simulink model "dSPACE_discrete"  (Simulink 7.1)
settings: Solver=ode3  StartTime=0.0  StopTime=inf  FixedStep=0.0005  RelTol=1e-3
undefined symbols (not defined in the file): DiscIntNeverNeededParam
libraries: simulink x2
settings Model: Creator=Administrator  LastModifiedBy=Administrator

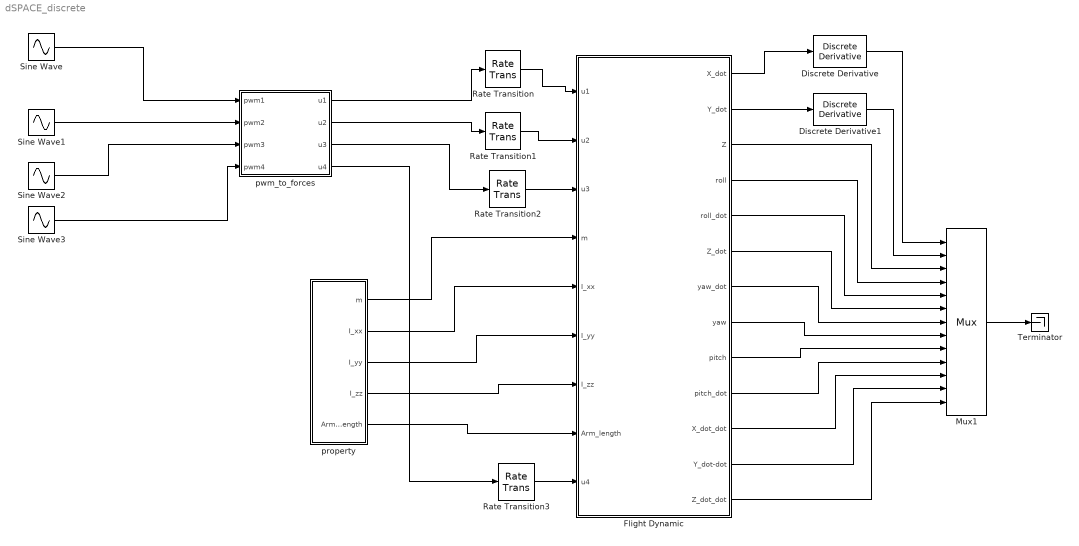
== system dSPACE_discrete ==
  Discrete Derivative : simulink/Discrete/Discrete Derivative  SystemSampleTime=-1  gainval=1.0  ICPrevScaledInput=0.0  OutMin=[]  OutMax=[]  OutDataType=sfix(16)  OutScaling=2^-10  DoSatur=off
  Discrete Derivative1 : simulink/Discrete/Discrete Derivative  SystemSampleTime=-1  gainval=1.0  ICPrevScaledInput=0.0  OutMin=[]  OutMax=[]  OutDataType=sfix(16)  OutScaling=2^-10  DoSatur=off
  Flight Dynamic : Subsystem
  Mux1 : Mux  Inputs=13
  Rate Transition{,1..3} (4 alike) : RateTransition
  Sine Wave{,1..3} (4 alike) : Sin  Amplitude=500  Bias=1500  SampleTime=0
  Terminator : Terminator
  "property " : Subsystem
  pwm_to_forces : Subsystem
  wires:
  Sine Wave1/1 -> pwm_to_forces/2(pwm2)
  Sine Wave2/1 -> pwm_to_forces/3(pwm3)
  Sine Wave3/1 -> pwm_to_forces/4(pwm4)
  Sine Wave/1 -> pwm_to_forces/1(pwm1)
  pwm_to_forces/1(u1) -> Rate Transition/1
  pwm_to_forces/2(u2) -> Rate Transition1/1
  pwm_to_forces/3(u3) -> Rate Transition2/1
  pwm_to_forces/4(u4) -> Rate Transition3/1
  "property "/1(m) -> Flight Dynamic/4(m)
  "property "/2(I_xx) -> Flight Dynamic/5(I_xx)
  "property "/3(I_yy) -> Flight Dynamic/6(I_yy)
  "property "/4(I_zz) -> Flight Dynamic/7(I_zz)
  "property "/5("Arm_length ") -> Flight Dynamic/8(Arm_length)
  Rate Transition/1 -> Flight Dynamic/1(u1)
  Rate Transition2/1 -> Flight Dynamic/3(u3)
  Rate Transition3/1 -> Flight Dynamic/9(u4)
  Rate Transition1/1 -> Flight Dynamic/2(u2)
  Flight Dynamic/1("X_dot ") -> Discrete Derivative/1
  Flight Dynamic/2(Y_dot) -> Discrete Derivative1/1
  Discrete Derivative/1 -> Mux1/1
  Discrete Derivative1/1 -> Mux1/2
  Flight Dynamic/3(Z) -> Mux1/3
  Flight Dynamic/4(roll) -> Mux1/4
  Flight Dynamic/5(roll_dot) -> Mux1/5
  Flight Dynamic/6(Z_dot) -> Mux1/6
  Flight Dynamic/7(yaw_dot) -> Mux1/7
  Flight Dynamic/8(yaw) -> Mux1/8
  Flight Dynamic/9(pitch) -> Mux1/9
  Flight Dynamic/10(pitch_dot) -> Mux1/10
  Flight Dynamic/11(X_dot_dot) -> Mux1/11
  Flight Dynamic/12(Y_dot-dot) -> Mux1/12
  Flight Dynamic/13(Z_dot_dot) -> Mux1/13
  Mux1/1 -> Terminator/1

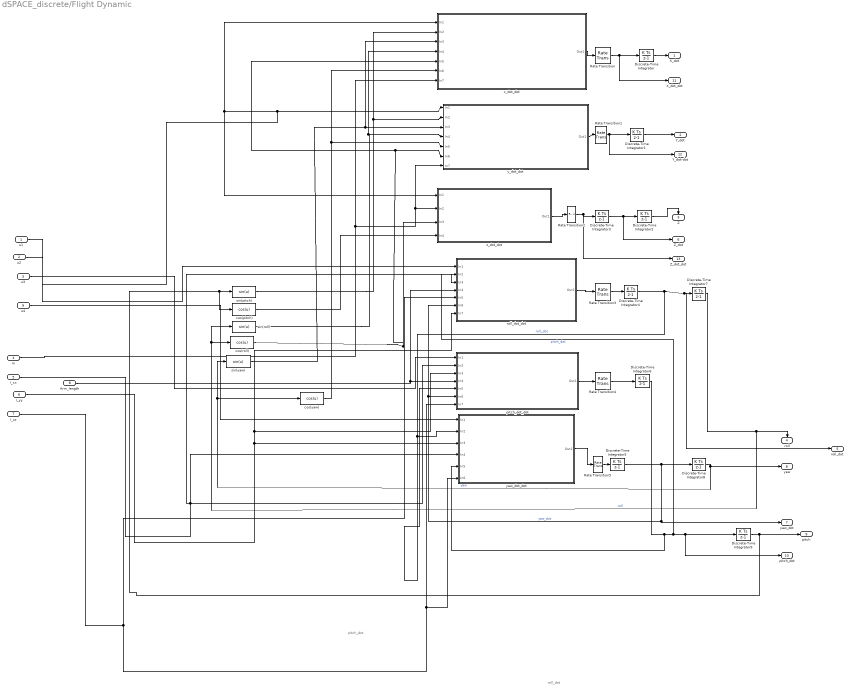
== system dSPACE_discrete/Flight Dynamic ==
  note: pitch_dot
  note: roll_dot
  u1 : Inport  OutDataType=sfix(16)  OutScaling=2^0
  u2 : Inport  Port=2  OutDataType=sfix(16)  OutScaling=2^0
  u3 : Inport  Port=3  OutDataType=sfix(16)  OutScaling=2^0
  m : Inport  Port=4  OutDataType=sfix(16)  OutScaling=2^0
  I_xx : Inport  Port=5  OutDataType=sfix(16)  OutScaling=2^0
  I_yy : Inport  Port=6  OutDataType=sfix(16)  OutScaling=2^0
  I_zz : Inport  Port=7  OutDataType=sfix(16)  OutScaling=2^0
  Arm_length : Inport  Port=8  OutDataType=sfix(16)  OutScaling=2^0
  u4 : Inport  Port=9  OutDataType=sfix(16)  OutScaling=2^0
  Discrete-Time Integrator{,1..9} (10 alike) : DiscreteIntegrator  OutDataType=sfix(16)  OutScaling=2^0  ICPrevOutput=DiscIntNeverNeededParam  ICPrevScaledInput=DiscIntNeverNeededParam
  Rate Transition{,1..5} (6 alike) : RateTransition
  cos(pitch) : Fcn  Expr=cos(u)
  cos(roll) : Fcn  Expr=cos(u)
  cos(yaw) : Fcn  Expr=cos(u)
  pitch_dot_dot : Subsystem
  roll_dot_dot : Subsystem
  sin(pitch) : Fcn  Expr=sin(u)
  sin(roll) : Fcn  Expr=sin(u)
  sin(yaw) : Fcn  Expr=sin(u)
  x_dot_dot : Subsystem
  y_dot_dot : Subsystem
  yaw_dot_dot : Subsystem
  z_dot_dot : Subsystem
  "X_dot " : Outport
  Y_dot : Outport  Port=2
  Z : Outport  Orientation=down  Port=3
  roll : Outport  Orientation=down  Port=4
  roll_dot : Outport  Port=5
  Z_dot : Outport  Port=6
  yaw_dot : Outport  Port=7
  yaw : Outport  Port=8
  pitch : Outport  Port=9
  pitch_dot : Outport  Port=10
  X_dot_dot : Outport  Port=11
  Y_dot-dot : Outport  Port=12
  Z_dot_dot : Outport  Port=13
  wires:
  x_dot_dot/1(Out1) -> Rate Transition/1
  Discrete-Time Integrator3/1 -> Z_dot/1, Discrete-Time Integrator2/1
  Discrete-Time Integrator7/1 -> roll/1, sin(roll)/1, cos(roll)/1  "roll"
  Discrete-Time Integrator6/1 -> yaw_dot_dot/5(In5), roll_dot_dot/2(In2), pitch_dot/1, Discrete-Time Integrator9/1  "pitch_dot"
  Discrete-Time Integrator5/1 -> roll_dot_dot/6(In6), pitch_dot_dot/6(In6), yaw_dot/1, Discrete-Time Integrator8/1  "yaw_dot"
  Discrete-Time Integrator4/1 -> pitch_dot_dot/5(In5), yaw_dot_dot/2(In2), roll_dot/1, Discrete-Time Integrator7/1  "roll_dot"
  Discrete-Time Integrator/1 -> "X_dot "/1
  Discrete-Time Integrator1/1 -> Y_dot/1
  Discrete-Time Integrator8/1 -> yaw/1, sin(yaw)/1, cos(yaw)/1  "yaw"
  z_dot_dot/1(Out1) -> Rate Transition2/1
  roll_dot_dot/1(Out1) -> Rate Transition3/1
  pitch_dot_dot/1(Out1) -> Rate Transition4/1
  y_dot_dot/1(Out1) -> Rate Transition1/1
  Discrete-Time Integrator9/1 -> pitch/1, sin(pitch)/1, cos(pitch)/1
  Discrete-Time Integrator2/1 -> Z/1
  yaw_dot_dot/1(Out1) -> Rate Transition5/1
  u4/1 -> yaw_dot_dot/1(In1)
  m/1 -> x_dot_dot/7(In7), z_dot_dot/2(In2), y_dot_dot/7(In7)
  u1/1 -> y_dot_dot/1(In1), x_dot_dot/1(In1), z_dot_dot/1(In1)
  I_xx/1 -> yaw_dot_dot/4(In4), roll_dot_dot/3(In3), pitch_dot_dot/2(In2)
  I_yy/1 -> yaw_dot_dot/3(In3), roll_dot_dot/7(In7), pitch_dot_dot/3(In3)
  I_zz/1 -> roll_dot_dot/5(In5), yaw_dot_dot/6(In6), pitch_dot_dot/7(In7)
  u2/1 -> roll_dot_dot/1(In1)
  Arm_length/1 -> roll_dot_dot/4(In4), pitch_dot_dot/4(In4)
  u3/1 -> pitch_dot_dot/1(In1)
  sin(pitch)/1 -> x_dot_dot/2(In2), y_dot_dot/2(In2)
  cos(pitch)/1 -> z_dot_dot/4(In4)
  sin(roll)/1 -> x_dot_dot/4(In4), y_dot_dot/4(In4)
  sin(yaw)/1 -> x_dot_dot/3(In3), y_dot_dot/3(In3)
  cos(yaw)/1 -> y_dot_dot/5(In5), x_dot_dot/6(In6)
  cos(roll)/1 -> x_dot_dot/5(In5), y_dot_dot/6(In6), z_dot_dot/3(In3)
  Rate Transition/1 -> X_dot_dot/1, Discrete-Time Integrator/1
  Rate Transition1/1 -> Y_dot-dot/1, Discrete-Time Integrator1/1
  Rate Transition3/1 -> Discrete-Time Integrator4/1
  Rate Transition4/1 -> Discrete-Time Integrator6/1
  Rate Transition5/1 -> Discrete-Time Integrator5/1
  Rate Transition2/1 -> Discrete-Time Integrator3/1, Z_dot_dot/1

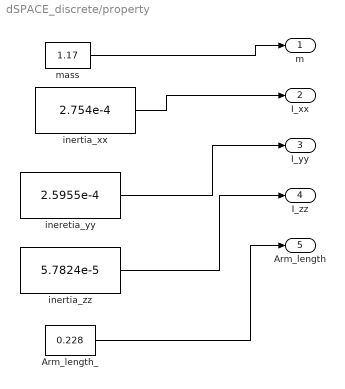
== system dSPACE_discrete/property  ==
  Arm_length_ : Constant  Value=0.228
  ineretia_yy : Constant  Value=2.5955e-4
  inertia_xx : Constant  Value=2.754e-4
  inertia_zz : Constant  Value=5.7824e-5
  mass : Constant  Value=1.17
  m : Outport
  I_xx : Outport  Port=2
  I_yy : Outport  Port=3
  I_zz : Outport  Port=4
  "Arm_length " : Outport  Port=5
  wires:
  inertia_zz/1 -> I_zz/1
  Arm_length_/1 -> "Arm_length "/1
  ineretia_yy/1 -> I_yy/1
  mass/1 -> m/1
  inertia_xx/1 -> I_xx/1

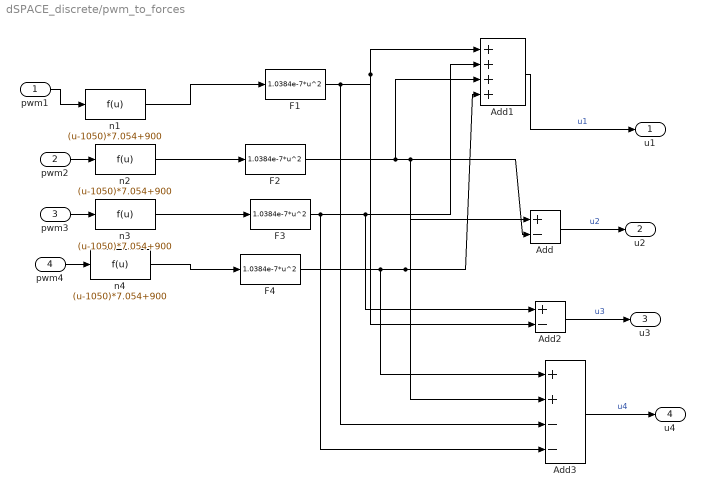
== system dSPACE_discrete/pwm_to_forces ==
  pwm1 : Inport
  pwm2 : Inport  Port=2
  pwm3 : Inport  Port=3
  pwm4 : Inport  Port=4
  Add : Sum  Inputs=+-  OutDataType=sfix(16)  OutScaling=2^-10
  Add1 : Sum  Inputs=++++  OutDataType=sfix(16)  OutScaling=2^-10
  Add2 : Sum  Inputs=+-  OutDataType=sfix(16)  OutScaling=2^-10
  Add3 : Sum  Inputs=++--  OutDataType=sfix(16)  OutScaling=2^-10
  F{1..4} (4 alike) : Fcn  Expr=1.0384e-7*u^2
  n{1..4} (4 alike) : Fcn  Expr=(u-1050)*7.054+900
  u1 : Outport  OutDataType=sfix(16)  OutScaling=2^0
  u2 : Outport  Port=2  OutDataType=sfix(16)  OutScaling=2^0
  u3 : Outport  Port=3  OutDataType=sfix(16)  OutScaling=2^0
  u4 : Outport  Port=4  OutDataType=sfix(16)  OutScaling=2^0
  wires:
  n1/1 -> F1/1
  n2/1 -> F2/1
  n3/1 -> F3/1
  n4/1 -> F4/1
  F1/1 -> Add1/1, Add2/2, Add3/3
  F2/1 -> Add1/3, Add/2, Add3/2
  F3/1 -> Add1/2, Add2/1, Add3/4
  F4/1 -> Add/1, Add1/4, Add3/1
  Add1/1 -> u1/1  "u1"
  Add/1 -> u2/1  "u2"
  Add2/1 -> u3/1  "u3"
  Add3/1 -> u4/1  "u4"
  pwm1/1 -> n1/1
  pwm2/1 -> n2/1
  pwm3/1 -> n3/1
  pwm4/1 -> n4/1

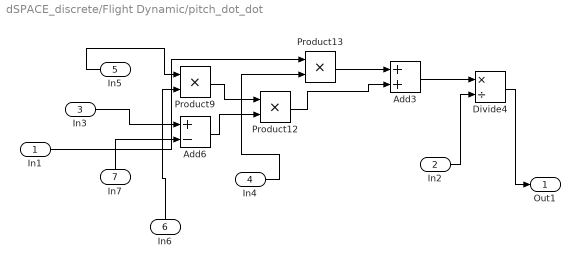
== system dSPACE_discrete/Flight Dynamic/pitch_dot_dot ==
  In1 : Inport
  In2 : Inport  Port=2
  In3 : Inport  Port=3
  In4 : Inport  Port=4
  In5 : Inport  Orientation=left  Port=5
  In6 : Inport  Orientation=up  Port=6
  In7 : Inport  Orientation=up  Port=7
  Add3 : Sum
  Add6 : Sum  Inputs=+-
  Divide4 : Product  Inputs=*/
  Product12 : Product
  Product13 : Product
  Product9 : Product
  Out1 : Outport
  wires:
  Product12/1 -> Add3/2
  Product13/1 -> Add3/1
  In1/1 -> Product13/1
  Add6/1 -> Product12/2
  Add3/1 -> Divide4/1
  Product9/1 -> Product12/1
  In4/1 -> Product13/2
  In6/1 -> Product9/2
  In7/1 -> Add6/2
  In3/1 -> Add6/1
  In2/1 -> Divide4/2
  In5/1 -> Product9/1
  Divide4/1 -> Out1/1

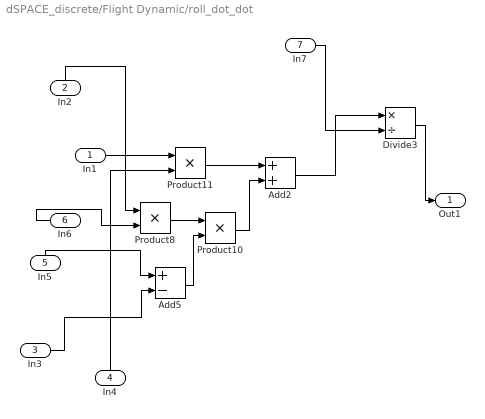
== system dSPACE_discrete/Flight Dynamic/roll_dot_dot ==
  In1 : Inport
  In2 : Inport  Orientation=up  Port=2
  In3 : Inport  Port=3
  In4 : Inport  Orientation=up  Port=4
  In5 : Inport  Orientation=up  Port=5
  In6 : Inport  Orientation=left  Port=6
  In7 : Inport  Port=7
  Add2 : Sum
  Add5 : Sum  Inputs=+-
  Divide3 : Product  Inputs=*/
  Product10 : Product
  Product11 : Product
  Product8 : Product
  Out1 : Outport
  wires:
  Product11/1 -> Add2/1
  Add5/1 -> Product10/2
  In1/1 -> Product11/1
  Add2/1 -> Divide3/1
  Product8/1 -> Product10/1
  Product10/1 -> Add2/2
  Divide3/1 -> Out1/1
  In5/1 -> Add5/1
  In3/1 -> Add5/2
  In2/1 -> Product8/1
  In7/1 -> Divide3/2
  In4/1 -> Product11/2
  In6/1 -> Product8/2

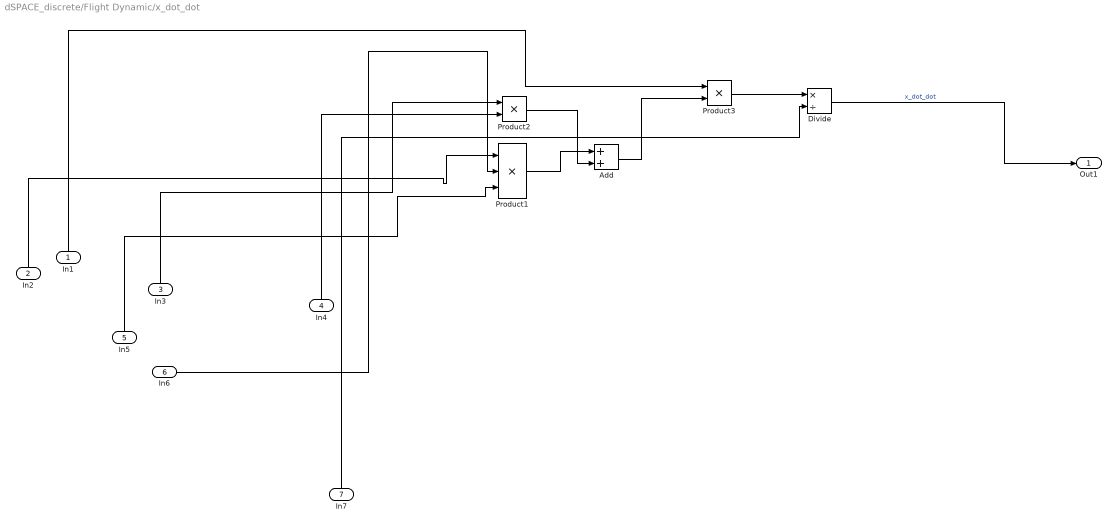
== system dSPACE_discrete/Flight Dynamic/x_dot_dot ==
  In1 : Inport  Orientation=up
  In2 : Inport  Orientation=up  Port=2
  In3 : Inport  Orientation=up  Port=3
  In4 : Inport  Orientation=up  Port=4
  In5 : Inport  Orientation=up  Port=5
  In6 : Inport  Port=6
  In7 : Inport  Orientation=up  Port=7
  Add : Sum
  Divide : Product  Inputs=*/
  Product1 : Product  Inputs=3
  Product2 : Product
  Product3 : Product
  Out1 : Outport
  wires:
  In1/1 -> Product3/1
  In6/1 -> Product1/2
  In7/1 -> Divide/2
  In4/1 -> Product2/2
  In3/1 -> Product2/1
  In5/1 -> Product1/3
  In2/1 -> Product1/1
  Divide/1 -> Out1/1  "x_dot_dot"
  Product2/1 -> Add/2
  Product1/1 -> Add/1
  Product3/1 -> Divide/1
  Add/1 -> Product3/2

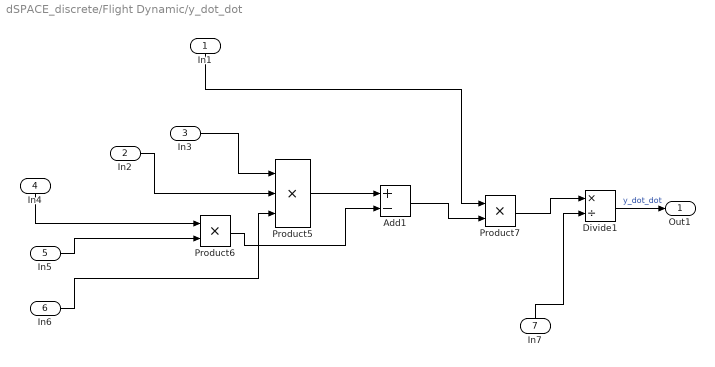
== system dSPACE_discrete/Flight Dynamic/y_dot_dot ==
  In1 : Inport  Orientation=down
  In2 : Inport  Port=2
  In3 : Inport  Port=3
  In4 : Inport  Orientation=down  Port=4
  In5 : Inport  Port=5
  In6 : Inport  Port=6
  In7 : Inport  Orientation=up  Port=7
  Add1 : Sum  Inputs=+-
  Divide1 : Product  Inputs=*/
  Product5 : Product  Inputs=3
  Product6 : Product
  Product7 : Product
  Out1 : Outport
  wires:
  In1/1 -> Product7/1
  In2/1 -> Product5/2
  In5/1 -> Product6/2
  In7/1 -> Divide1/2
  In6/1 -> Product5/3
  In3/1 -> Product5/1
  In4/1 -> Product6/1
  Product5/1 -> Add1/1
  Add1/1 -> Product7/2
  Product6/1 -> Add1/2
  Divide1/1 -> Out1/1  "y_dot_dot"
  Product7/1 -> Divide1/1

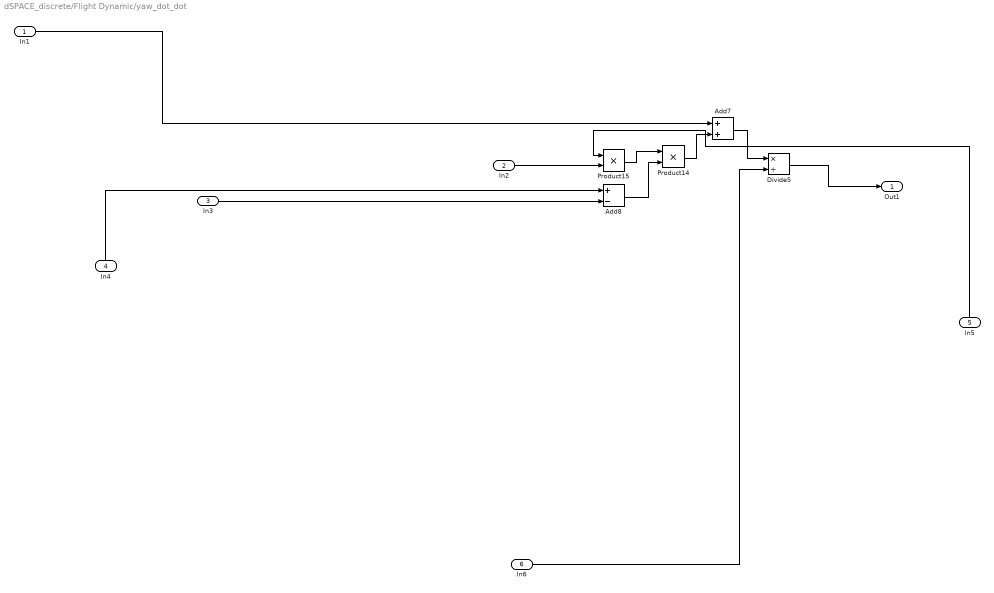
== system dSPACE_discrete/Flight Dynamic/yaw_dot_dot ==
  In1 : Inport
  In2 : Inport  Port=2
  In3 : Inport  Port=3
  In4 : Inport  Orientation=up  Port=4
  In5 : Inport  Orientation=up  Port=5
  In6 : Inport  Port=6
  Add7 : Sum
  Add8 : Sum  Inputs=+-
  Divide5 : Product  Inputs=*/
  Product14 : Product
  Product15 : Product
  Out1 : Outport
  wires:
  In4/1 -> Add8/1
  In6/1 -> Divide5/2
  In2/1 -> Product15/2
  In3/1 -> Add8/2
  In5/1 -> Product15/1
  Product14/1 -> Add7/2
  Add8/1 -> Product14/2
  Product15/1 -> Product14/1
  In1/1 -> Add7/1
  Add7/1 -> Divide5/1
  Divide5/1 -> Out1/1

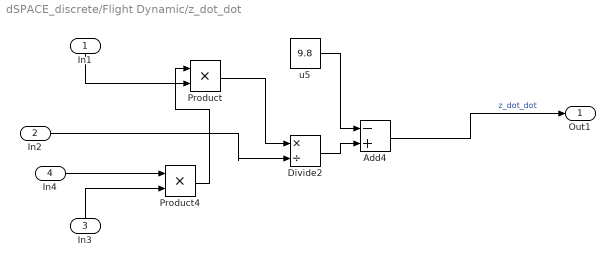
== system dSPACE_discrete/Flight Dynamic/z_dot_dot ==
  In1 : Inport  Orientation=down
  In2 : Inport  Port=2
  In3 : Inport  Orientation=up  Port=3
  In4 : Inport  Port=4
  Add4 : Sum  Inputs=-+
  Divide2 : Product  Inputs=*/
  Product : Product
  Product4 : Product
  u5 : Constant  Value=9.8
  Out1 : Outport
  wires:
  In3/1 -> Product4/2
  In2/1 -> Divide2/2
  In1/1 -> Product/2
  Divide2/1 -> Add4/2
  Product4/1 -> Product/1
  In4/1 -> Product4/1
  u5/1 -> Add4/1
  Product/1 -> Divide2/1
  Add4/1 -> Out1/1  "z_dot_dot"
